simulink model "matlab_table_2019b.slx"  (R2019b)
settings: Solver=FixedStepAuto  StartTime=0.0  StopTime=200  RelTol=1e-3  EnableMultiTasking=on
InitFcn:
  | simin.time = [];
  | simin.signals.values = [10:5:90]';
libraries: mbedblockslib x5
settings Model: SimulationMode=external  SILPILModeSetting=veronly  ExtModeTrigDuration=10  Creator=The MathWorks, Inc.  LastModifiedBy=User
settings SolverCC: PositivePriorityOrder=on
settings DataIOCC: ReturnWorkspaceOutputs=off
settings OptimizationCC: MaxStackSize=64
settings DebuggingCC: ParameterTunabilityLossMsg=error  ArithmeticOperatorsInVariantConditions=warning
settings HardwareCC: ProdBitPerPointer=32  ProdBitPerSizeT=32  ProdBitPerPtrDiffT=32  ProdLargestAtomicInteger=Long  ProdLargestAtomicFloat=Double  ProdWordSize=32  ProdHWDeviceType=ARM Compatible->ARM Cortex  UseEmbeddedCoderFeatures=off
settings ModelReferenceCC: ModelReferenceNumInstancesAllowed=Single
settings SFSimCC: SimUseLocalCustomCode=off  CustomCodeUndefinedFunction=UseInterfaceOnly
settings RTWCC: SystemTargetFile=ert.tlc  HardwareBoard=STM32 Nucleo F767ZI  TemplateMakefile=ert_default_tmf  GenerateReport=on  RTWUseLocalCustomCode=off  Toolchain=GNU Tools for ARM Embedded Processors  LaunchReport=on
settings CodeAppCC: ForceParamTrailComments=on  OperatorAnnotations=on  StateflowObjectComments=on  MATLABSourceComments=on
settings ERTTargetCC: CodeReplacementLibrary=ARM Cortex-M (Optimized)  MultiwordLength=2048  ERTCustomFileBanners=off  SupportContinuousTime=on  SupportNonInlinedSFcns=on  RemoveResetFunc=off  ModelStepFunctionPrototypeControlCompliant=off  ExtMode=on  ExtModeTransport=3  ExtModeStaticAlloc=on  ExtModeStaticAllocSize=2000  ExtModeMexFile=ext_xcp  ExtModeMexArgs=1 3 115200  ExtModeIntrfLevel=Level2 - Open  ERTSrcFileBannerTemplate=codertarget_code_template.cgt  ERTHdrFileBannerTemplate=codertarget_code_template.cgt  ERTDataSrcFileTemplate=codertarget_code_template.cgt  ERTDataHdrFileTemplate=codertarget_code_template.cgt
settings ConfigComp: CovMetricSettings=dsw  CovHtmlReporting=on  CovSaveCumulativeToWorkspaceVar=on  CovSaveSingleToWorkspaceVar=on  CovShowResultsExplorer=off  CovExternalEMLEnable=off

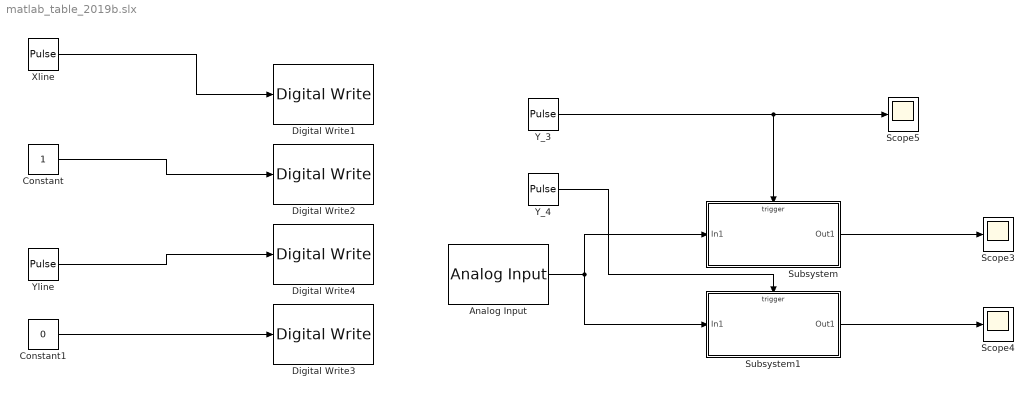
== system matlab_table_2019b.slx ==
  Analog Input : mbedblockslib/Analog Input  Pin=PC_3  ReadResultsOnly=off  ConversionTriggerSource=Software  ExternalTriggerType=uint32( 0 )  OutputDataType=double  EnableConversionCompleteNotify=off  EnableOuputStatus=off  SampleTime=-1
      settings: SourceProductName=Simulink Coder Support Package for BBC microbit Board  SourceProductBaseCode=MICROBIT
  Constant : Constant
  Constant1 : Constant  Value=0
  Digital Write1 : mbedblockslib/Digital Write  Pin=PD_6  Direction=output
      settings: SourceProductName=Simulink Coder Support Package for BBC microbit Board  SourceProductBaseCode=MICROBIT
  Digital Write2 : mbedblockslib/Digital Write  Pin=PD_5  Direction=output
      settings: SourceProductName=Simulink Coder Support Package for BBC microbit Board  SourceProductBaseCode=MICROBIT
  Digital Write3 : mbedblockslib/Digital Write  Pin=PD_3  Direction=output
      settings: SourceProductName=Simulink Coder Support Package for BBC microbit Board  SourceProductBaseCode=MICROBIT
  Digital Write4 : mbedblockslib/Digital Write  Pin=PD_4  Direction=output
      settings: SourceProductName=Simulink Coder Support Package for BBC microbit Board  SourceProductBaseCode=MICROBIT
  Scope3 : Scope
  Scope4 : Scope
  Scope5 : Scope
  Subsystem : Subsystem
  Subsystem1 : Subsystem
  Xline : DiscretePulseGenerator  PulseType=Time based  Period=500*10^(-6)  PulseWidth=50  PhaseDelay=250*10^(-6)
  Y_3 : DiscretePulseGenerator  PulseType=Time based  Period=500*10^(-6)  PhaseDelay=200*10^(-6)
  Y_4 : DiscretePulseGenerator  PulseType=Time based  Period=500*10^(-6)  PhaseDelay=450*10^(-6)
  "Yline " : DiscretePulseGenerator  PulseType=Time based  Period=500*10^(-6)  PulseWidth=50
  wires:
  Y_3/1 -> Subsystem/Trigger, Scope5/1
  Y_4/1 -> Subsystem1/Trigger
  Analog Input/1 -> Subsystem/1(In1), Subsystem1/1(In1)
  Subsystem1/1(Out1) -> Scope4/1
  Subsystem/1(Out1) -> Scope3/1
  Xline/1 -> Digital Write1/1
  Constant/1 -> Digital Write2/1
  "Yline "/1 -> Digital Write4/1
  Constant1/1 -> Digital Write3/1

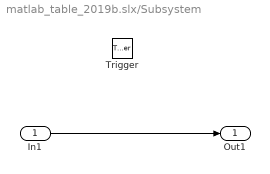
== system matlab_table_2019b.slx/Subsystem ==
  In1 : Inport
  Trigger : TriggerPort  VariantControl=Variant  PortDimensions=1
  Out1 : Outport
  wires:
  In1/1 -> Out1/1

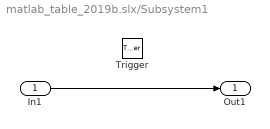
== system matlab_table_2019b.slx/Subsystem1 ==
  In1 : Inport
  Trigger : TriggerPort  VariantControl=Variant  PortDimensions=1
  Out1 : Outport
  wires:
  In1/1 -> Out1/1
